simulink model "BE_simu"  (R2018b)
settings: Solver=VariableStepAuto  StartTime=0.0  StopTime=10  RelTol=1e-3
settings Model: Creator=piffercg  LastModifiedBy=piffercg

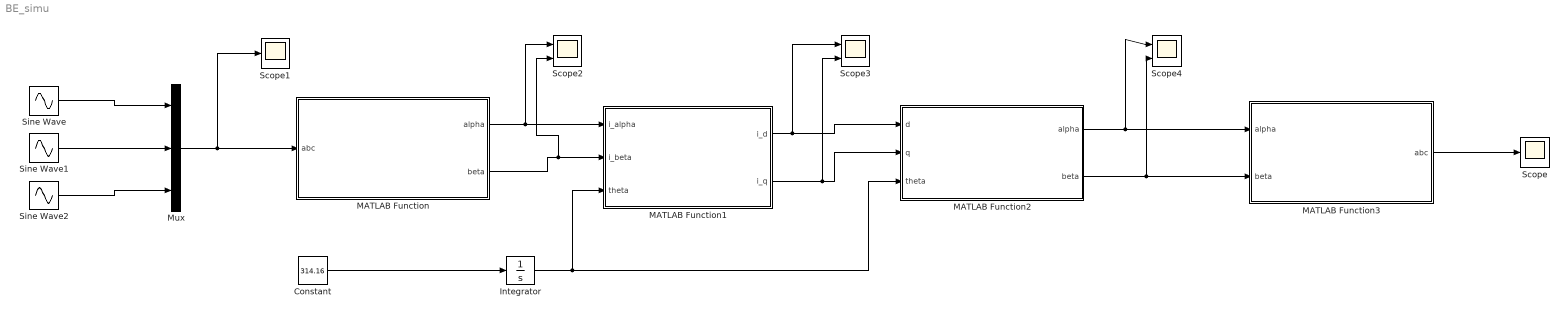
== system BE_simu ==
  Constant : Constant  Value=314.16
  Integrator : Integrator
  MATLAB Function : MATLAB Function  TreatAsAtomicUnit=on
  MATLAB Function1 : MATLAB Function  TreatAsAtomicUnit=on
  MATLAB Function2 : MATLAB Function  TreatAsAtomicUnit=on
  MATLAB Function3 : MATLAB Function  TreatAsAtomicUnit=on
  Mux : Mux  Inputs=3
  Scope : Scope
  Scope1 : Scope
  Scope2 : Scope  NumInputPorts=2
  Scope3 : Scope  NumInputPorts=2
  Scope4 : Scope  NumInputPorts=2
  Sine Wave : Sin  Amplitude=36  Frequency=314.16  SampleTime=0
  Sine Wave1 : Sin  Amplitude=36  Frequency=314.16  Phase=2*pi/3  SampleTime=0
  Sine Wave2 : Sin  Amplitude=36  Frequency=314.16  Phase=-2*pi/3  SampleTime=0
  wires:
  Sine Wave1/1 -> Mux/2
  Sine Wave2/1 -> Mux/3
  Sine Wave/1 -> Mux/1
  Mux/1 -> Scope1/1, MATLAB Function/1(abc)
  MATLAB Function/1(alpha) -> Scope2/1, MATLAB Function1/1(i_alpha)
  MATLAB Function/2(beta) -> Scope2/2, MATLAB Function1/2(i_beta)
  MATLAB Function1/1(i_d) -> Scope3/1, MATLAB Function2/1(d)
  MATLAB Function1/2(i_q) -> Scope3/2, MATLAB Function2/2(q)
  MATLAB Function2/1(alpha) -> Scope4/1, MATLAB Function3/1(alpha)
  MATLAB Function2/2(beta) -> Scope4/2, MATLAB Function3/2(beta)
  MATLAB Function3/1(abc) -> Scope/1
  Integrator/1 -> MATLAB Function2/3(theta), MATLAB Function1/3(theta)
  Constant/1 -> Integrator/1

== matlab function BE_simu/MATLAB Function1 ==
  data: i_alpha input; i_d output; i_beta input; theta input; i_q output
function [i_d,i_q] = Park(i_alpha,i_beta,theta)
i_d = i_alpha*cos(theta)+i_beta*sin(theta);
i_q = -i_alpha*sin(theta)+i_beta*cos(theta);
end

== matlab function BE_simu/MATLAB Function ==
  data: abc input; alpha output; beta output
function [alpha, beta] = transformClarke(abc)
    T_clarke = sqrt(2/3) * [1 -1/2 -1/2; 0 sqrt(3)/2 -sqrt(3)/2];
    alpha_beta = T_clarke * abc;
    
    alpha = alpha_beta(1);
    beta = alpha_beta(2);
end

== matlab function BE_simu/MATLAB Function2 ==
  data: d input; alpha output; q input; theta input; beta output
function [alpha, beta] = transformInvPark(d, q, theta)
    T_park_inv = [cos(theta), sin(theta); -sin(theta), cos(theta)];
    
    dq = [d; q];
    alpha_beta = T_park_inv * dq;
    
    alpha = alpha_beta(1);
    beta = alpha_beta(2);
end

== matlab function BE_simu/MATLAB Function3 ==
  data: alpha input; abc output; beta input
function abc  = transformInvClarke(alpha, beta)
    T_clarke_inv = sqrt(2/3) * [1, 0; -1/2, sqrt(3)/2; -1/2, -sqrt(3)/2];
    
    alpha_beta = [alpha; beta];
    abc = T_clarke_inv * alpha_beta;
end
